simulink model "LQG_integral_action"  (R2022b)
settings: Solver=VariableStepAuto  StartTime=0.0  StopTime=60  RelTol=1e-3
values from neighbouring files (symbols this model uses):
  Ad = [0.401010357696 0.207607414378 0.0585143980091 -782.832786661 342.529887341 0.596372065474 0.774865707155 0.568579797376 773.747483889 -370.95887721 0.00261757683024 0.0175268784671 ... (25 elements, 5x5)]    [A_d.mat]    (also in ref.m = expm(Av*Ts))
  Bd = [0.00315440131404  0.000285742610066; 0.000159453102519  0.00321146251052; 2.85742610066e-05  0.316758560203; 4.4993079134  1.30878841512; 0.585143980091  8.76343923355]    [B_d.mat]    (also in ref.m = double(int(exp_At,t,0,Ts)*Bv))
  C1 = [0  1  0  0  0; 0  0  0  0  1]    [C.mat]    (also in ref.m = jacobian(x(:,1), [phi2(1);w2(1)]).')
  D_1 = [0  0; 0  0]    [D.mat]
  K_I = K2(:,6)*150    [Assignment3.m]    (also in ref.m = Klqr(:,length(Ad)+1:end)*20)
  K_p = K2(:,1:5)    [Assignment3.m]
undefined symbols (not defined in the file or in its folder): DiscIntNeverNeededParam, L
settings Model: Creator=Yogith  LastModifiedBy=aksha
settings DebuggingCC: UnconnectedInputMsg=warning  UnconnectedOutputMsg=warning  UnconnectedLineMsg=warning
settings ModelReferenceCC: EnableRefExpFcnMdlSchedulingChecks=on
settings RTWCC: DLArmComputeVersion=19.05

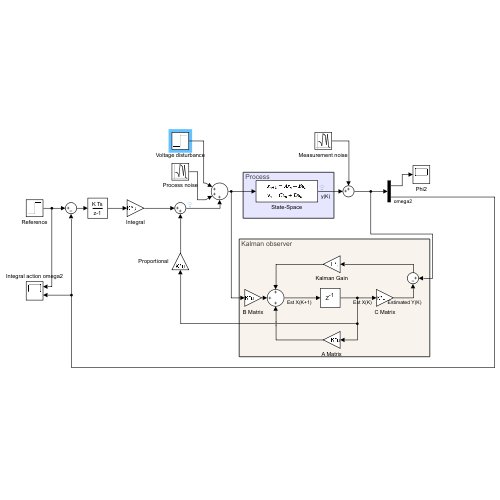
[thumbnail: Simulink's stored preview of the top-level diagram]
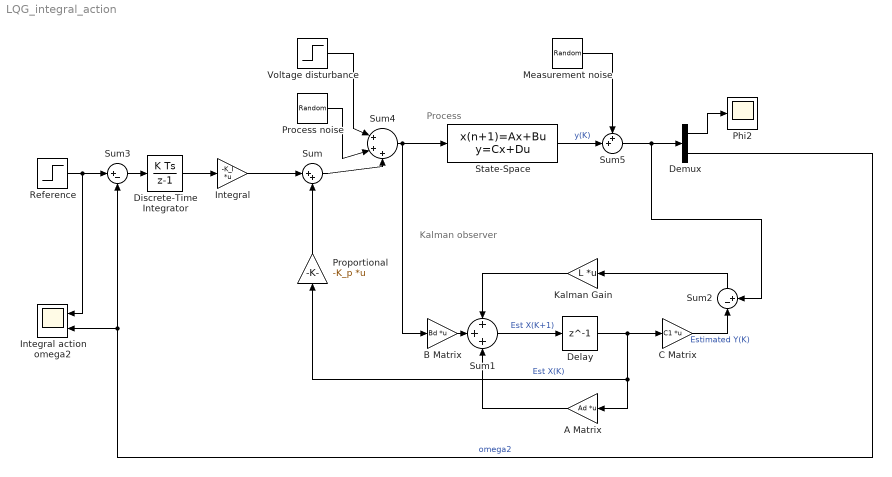
== system LQG_integral_action ==
  note: Process
  note: Kalman observer
  A Matrix : Gain  Gain=Ad  Multiplication=Matrix(K*u)
  B Matrix : Gain  Gain=Bd  Multiplication=Matrix(K*u)
  C Matrix : Gain  Gain=C1  Multiplication=Matrix(K*u)
  Delay : Delay  DelayLength=1
  Demux : Demux  Outputs=2
  Discrete-Time Integrator : DiscreteIntegrator  SampleTime=-1  ICPrevOutput=DiscIntNeverNeededParam  ICPrevScaledInput=DiscIntNeverNeededParam
  Integral : Gain  Gain=-K_I  Multiplication=Matrix(K*u)
  Integral action omega2 : Scope  NumInputPorts=2
  Kalman Gain : Gain  Gain=L  Multiplication=Matrix(K*u)
  Measurement noise : RandomNumber  Variance=[(0.02/3)^2 ; (0.01/3)^2]  SampleTime=0.1
  Phi2 : Scope
  Process noise : RandomNumber  Variance=[(0.3/3)^2; (0.1/3)^2]  SampleTime=0.1
  Proportional : Gain  Gain=-K_p  Multiplication=Matrix(K*u)
  Reference : Step  Time=10  Before=10  After=100  SampleTime=0
  State-Space : DiscreteStateSpace  A=Ad  B=Bd  C=C1  D=D_1  SampleTime=-1  StateName=sys_extend
  Sum : Sum  Inputs=|++
  Sum1 : Sum  Inputs=+++
  Sum2 : Sum  Inputs=|-+
  Sum3 : Sum  Inputs=|+-
  Sum4 : Sum  Inputs=|+++
  Sum5 : Sum  Inputs=++|
  Voltage disturbance : Step  Time=5  SampleTime=0
  wires:
  Demux/1 -> Phi2/1
  Demux/2 -> Sum3/2, Integral action omega2/2  "omega2"
  Sum/1 -> Sum4/3
  B Matrix/1 -> Sum1/2
  Sum1/1 -> Delay/1  "Est X(K+1)"
  Kalman Gain/1 -> Sum1/1
  Delay/1 -> A Matrix/1, Proportional/1, C Matrix/1  "Est X(K)"
  C Matrix/1 -> Sum2/1  "Estimated Y(K)"
  Sum2/1 -> Kalman Gain/1
  A Matrix/1 -> Sum1/3
  Proportional/1 -> Sum/2
  Reference/1 -> Integral action omega2/1, Sum3/1
  Integral/1 -> Sum/1
  Sum5/1 -> Sum2/2, Demux/1
  Sum3/1 -> Discrete-Time Integrator/1
  Discrete-Time Integrator/1 -> Integral/1
  Sum4/1 -> B Matrix/1, State-Space/1
  Process noise/1 -> Sum4/2
  Voltage disturbance/1 -> Sum4/1
  State-Space/1 -> Sum5/2  "y(K)"
  Measurement noise/1 -> Sum5/1
